simulink model "arithmetic"  (R2025a)
settings: Solver=FixedStepAuto  StartTime=0.0  StopTime=5  FixedStep=0.00001  MaxStep=0.001  RelTol=1e-3
values from neighbouring files (symbols this model uses):
  Fx = 600.0    [data.sldd]    (also in data2023.sldd)
  Fy = 800.0    [data.sldd]    (also in data2023.sldd)
  g = 10.0    [data.sldd]    (also in data2023.sldd)
  ma = 20.0    [data.sldd]    (also in data2023.sldd)
  mb = 50.0    [data.sldd]    (also in data2023.sldd)
  T0 = 500.0    [data.sldd]    (also in data2023.sldd = 20.0)
settings Model: DataDictionary=data.sldd  Creator=MangoJuice  LastModifiedBy=MangoJuice

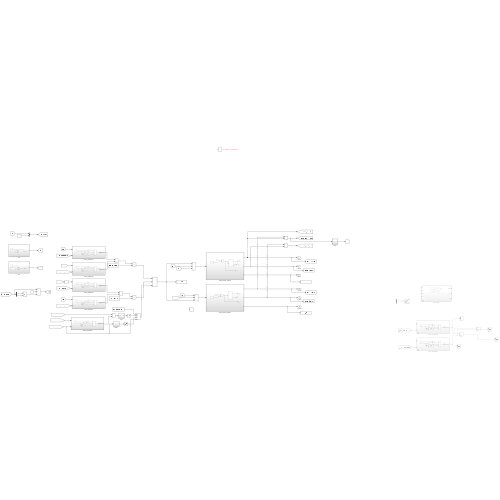
[thumbnail: Simulink's stored preview of the top-level diagram]
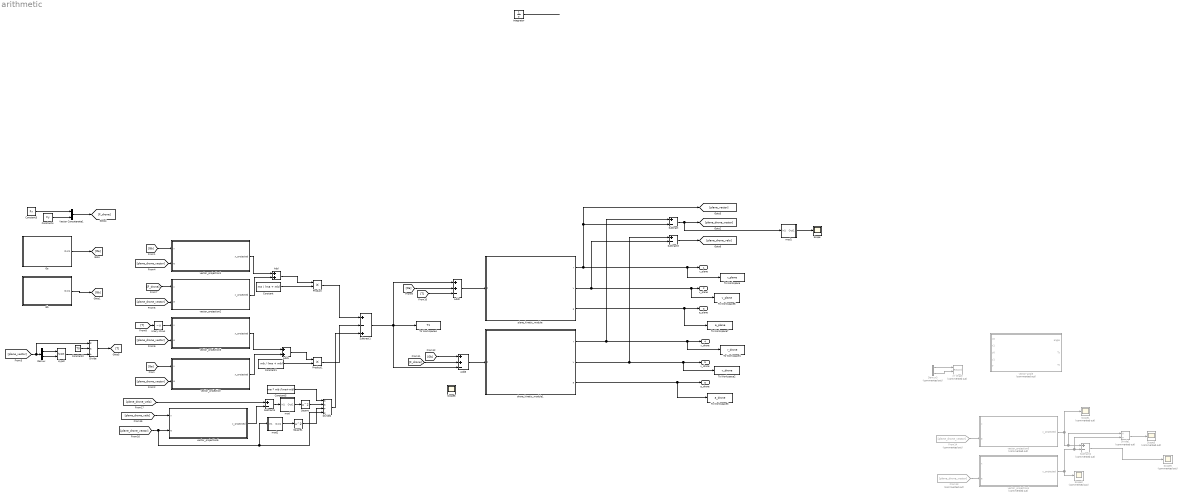
== system arithmetic ==
  Add : Sum
  Add1 : Sum
  Add2 : Sum  Inputs=++-
  Add3 : Sum  Inputs=++-
  Constant : Constant  Value=ma / (ma + mb)
  Constant1 : Constant  Value=mb / (ma + mb)
  Constant2 : Constant  Value=T0
  Constant3 : Constant  Value=Fx
  Constant4 : Constant  Value=Fy
  Constant5 : Constant  Value=ma * mb /(ma+mb)
  Demux : Demux  Outputs=2
  Demux3 : Demux  Commented=on  Outputs=2
  Divide : Product  Inputs=**/
  Divide1 : Product  Commented=on  Inputs=*/
  Divide2 : Product  Inputs=**/*
  From13 : From  Commented=on  GotoTag=plane_drone_vector
  From14 : From  Commented=on  GotoTag=plane_drone_vector
  Ga : Subsystem
  Gb : Subsystem
  Hypot : Math  Operator=hypot
  Integrator : Integrator
  Product : Product
  Product1 : Product
  Scope : Scope
      settings: ActiveDisplayYMinimum=49.999999999997144  ActiveDisplayYMaximum=50.0000000000041
  Scope{1..3,5} (4 alike) : Scope  Commented=on
      Scope1 settings: ActiveDisplayYMinimum=-1.094437041420969  ActiveDisplayYMaximum=6.4337390050976033
      Scope2 settings: ActiveDisplayYMinimum=-1  ActiveDisplayYMaximum=1  DataLoggingVariableName=ScopeData2
      Scope3 settings: ActiveDisplayYMinimum=-1.2740170172523153  ActiveDisplayYMaximum=0.9918630866201682  DataLoggingVariableName=ScopeData3
      Scope5 settings: ActiveDisplayYMinimum=-10.22400956516295  ActiveDisplayYMaximum=15.11556177661943  DataLoggingVariableName=ScopeData5
  Scope6 : Scope
      settings: ActiveDisplayYMinimum=99.999999999999943  ActiveDisplayYMaximum=100.00000000000006  DataLoggingVariableName=ScopeData6
  Square : Math  Operator=square
  Square1 : Math  Operator=square
  Subtract : Sum  Inputs=+-
  Subtract1 : Sum  Inputs=+-+
  Subtract2 : Sum  Commented=on  Inputs=+-
  Subtract3 : Sum  Inputs=+-
  Subtract4 : Sum  Inputs=+-
  To Workspace : ToWorkspace  VariableName=r_plane  SaveFormat=Timeseries  SampleTime=0.05
  To Workspace1 : ToWorkspace  VariableName=r_drone  SaveFormat=Timeseries  SampleTime=0.05
  To Workspace2 : ToWorkspace  VariableName=v_drone  SaveFormat=Timeseries  SampleTime=0.05
  To Workspace3 : ToWorkspace  VariableName=a_drone  SaveFormat=Timeseries  SampleTime=0.05
  To Workspace4 : ToWorkspace  VariableName=T1  SaveFormat=Timeseries  SampleTime=0.05
  To Workspace6 : ToWorkspace  VariableName=v_plane  SaveFormat=Timeseries  SampleTime=0.05
  To Workspace7 : ToWorkspace  VariableName=a_plane  SaveFormat=Timeseries  SampleTime=0.05
  Unary Minus : UnaryMinus
  Vector Concatenate1 : Concatenate
  XY Graph : Record  Commented=on  NumPorts=2.0  FileSettingsInternal="{\"entries\":[{\"content\":{\"excelSettings\":{\"content\":{},\"type\":\"Streamout.ExcelSettings\"},\"parquetSettings\":{\"content\":{},\"type\":\"Streamout.ParquetSettings\"}},\"type\":\"Streamout.FileSettingStorage\",\"uuid\":\"\"}],\"packageUris\":[\"http:\\/\\/schema.mathworks.com\\/mf0\\/streamout_blocks\\/R2020a\"],\"version\":\"1.0\"}"  FrameSettings=[0, 0]  Layout=[1 1]  SignalsInternal="{\"entries\":[{\"content\":{\"signals\":[{\"content\":{\"blockPath\":[],\"dimensions\":[1],\"domain\":\"\",\"lineColor\":\"#a2142f\",\"plots\":[ 1 ],\"port\":1,\"sid\":[\"\"],\"signalID\":1,\"signalName\":\"Demux3:1\"},\"type\":\"RecordBlkView.Signal\",\"uuid\":\"\"},{\"content\":{\"blockPath\":[],\"dimensions\":[1],\"domain\":\"\",\"lineColor\":\"#139fff\",\"plots\":[ 1 ],\"port\":2,\"sid\":[\"\"],\"signalID\":2,\"signalName\":\"Demux3:2\"},\"type\":\"RecordBlkView.Signal\",\"uuid\":\"\"}]},\"type\":\"RecordBlkView.InputSignals\",\"uuid\":\"\"}],\"packageUris\":[\"http:\\/\\/schema.mathworks.com\\/mf0\\/streamout_blocks\\/R2020a\"],\"version\":\"1.0\"}"  VisualizationBindings="{\"xyplotplugin\":{\"info\":[{\"series\":[{\"bindingParametersList\":[{\"parameter\":\"X-Axis\",\"signalID\":1,\"signalName\":\"Demux3:1\"},{\"parameter\":\"Y-Axis\",\"signalID\":2,\"signalName\":\"Demux3:2\"}],\"seriesID\":0}],\"subplotID\":1}]}}"  CompatibilityTag=XY
  drone_kinetic_module1 : Subsystem
  mod : Subsystem
  mod1 : Subsystem
  mod2 : Subsystem
  plane_kinetic_module : Subsystem
  vector-angle : Subsystem  Commented=on
  vector_projection : Subsystem
  vector_projection1 : Subsystem
  vector_projection2 : Subsystem
  vector_projection3 : Subsystem
  vector_projection4 : Subsystem  Commented=on
  vector_projection5 : Subsystem  Commented=on
  vector_projection6 : Subsystem
  r_plane : Outport
  v_plane : Outport  Port=2
  a_plane : Outport  Port=3
  r_drone : Outport  Port=4
  v_drone : Outport  Port=5
  a_drone : Outport  Port=6
  wires:
  Integrator/1 -> ?
  Ga/1(Out1) -> [Ga]
  Gb/1(Out1) -> [Gb]
  plane_kinetic_module/1(r) -> To Workspace/1, r_plane/1, [plane_vector], Subtract/2
  Subtract/1 -> mod1/1(In1), [plane_drone_vector]
  Hypot/1 -> Divide/3
  [plane_vector] -> Divide/1, Demux/1
  Demux/2 -> Hypot/2
  Demux/1 -> Hypot/1
  Constant2/1 -> Divide/2
  Vector Concatenate1/1 -> [F_drone]
  Constant3/1 -> Vector Concatenate1/1
  Constant4/1 -> Vector Concatenate1/2
  [Ga] -> vector_projection/1(x)
  [Gb] -> vector_projection1/1(x)
  [F_drone] -> vector_projection2/1(x)
  [plane_drone_vector] -> vector_projection/2(e)
  [plane_drone_vector] -> vector_projection1/2(e)
  [plane_drone_vector] -> vector_projection2/2(e)
  [plane_drone_vector] -> vector_projection3/2(e)
  vector_projection1/1(x_projected) -> Add/1
  vector_projection2/1(x_projected) -> Add/2
  Add/1 -> Product/1
  vector_projection3/1(x_projected) -> Add1/1
  vector_projection/1(x_projected) -> Add1/2
  Add1/1 -> Product1/1
  Product/1 -> Subtract1/1
  Product1/1 -> Subtract1/2
  Constant/1 -> Product/2
  Constant1/1 -> Product1/2
  Subtract1/1 -> To Workspace4/1, Add3/3, Add2/1
  Add2/1 -> plane_kinetic_module/1(F)
  [Ga] -> Add2/2
  [T] -> Add2/3
  Add3/1 -> drone_kinetic_module1/1(F)
  [F_drone] -> Add3/2
  [Gb] -> Add3/1
  vector_projection5/1(x_projected) -> Scope1/1, Divide1/1, Subtract2/1
  vector_projection4/1(x_projected) -> Scope2/1, Divide1/2, Subtract2/2
  From14/1 -> vector_projection5/2(e)
  From13/1 -> vector_projection4/2(e)
  Demux3/2 -> XY Graph/2
  Demux3/1 -> XY Graph/1
  Divide/1 -> [T]
  [T] -> Unary Minus/1
  Unary Minus/1 -> vector_projection3/1(x)
  Subtract2/1 -> Scope5/1
  Divide1/1 -> Scope3/1
  Subtract3/1 -> [plane_drone_velo]
  drone_kinetic_module1/2(v) -> To Workspace2/1, v_drone/1, Subtract3/1
  [plane_drone_velo] -> vector_projection6/1(x)
  vector_projection6/1(x_projected) -> Subtract4/2
  [plane_drone_velo] -> Subtract4/1
  Subtract4/1 -> mod/1(In1)
  mod/1(Out1) -> Square/1
  mod2/1(Out1) -> Square1/1
  [plane_drone_vector] -> Divide2/4, mod2/1(In1), vector_projection6/2(e)
  Square/1 -> Divide2/2
  Square1/1 -> Divide2/3
  Divide2/1 -> Subtract1/3
  Constant5/1 -> Divide2/1
  plane_kinetic_module/3(a) -> To Workspace7/1, a_plane/1
  drone_kinetic_module1/3(a) -> To Workspace3/1, a_drone/1
  plane_kinetic_module/2(v) -> To Workspace6/1, v_plane/1, Subtract3/2
  drone_kinetic_module1/1(r) -> To Workspace1/1, r_drone/1, Subtract/1
  mod1/1(Out1) -> Scope/1

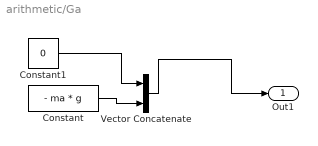
== system arithmetic/Ga ==
  Constant : Constant  Value=- ma * g  VectorParams1D=off
  Constant1 : Constant  Value=0
  Vector Concatenate : Concatenate
  Out1 : Outport
  wires:
  Constant1/1 -> Vector Concatenate/1
  Constant/1 -> Vector Concatenate/2
  Vector Concatenate/1 -> Out1/1

== system arithmetic/Gb ==
  Constant : Constant  Value=- mb * g  VectorParams1D=off
  Constant1 : Constant  Value=0
  Vector Concatenate : Concatenate
  Out1 : Outport
  wires:
  Vector Concatenate/1 -> Out1/1
  Constant/1 -> Vector Concatenate/2
  Constant1/1 -> Vector Concatenate/1

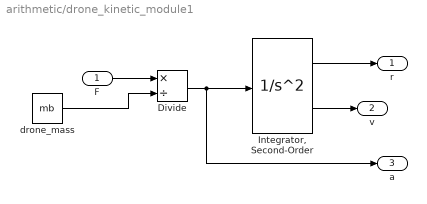
== system arithmetic/drone_kinetic_module1 ==
  F : Inport
  Divide : Product  Inputs=*/
  "Integrator, Second-Order" : SecondOrderIntegrator  ICX=drone_r0  ICDXDT=drone_v0
  drone_mass : Constant  Value=mb
  r : Outport
  v : Outport  Port=2
  a : Outport  Port=3
  wires:
  drone_mass/1 -> Divide/2
  "Integrator, Second-Order"/2 -> v/1
  "Integrator, Second-Order"/1 -> r/1
  Divide/1 -> a/1, "Integrator, Second-Order"/1
  F/1 -> Divide/1

== system arithmetic/mod ==
  In1 : Inport
  Demux4 : Demux  Outputs=2
  Hypot3 : Math  Operator=hypot
  Out1 : Outport
  wires:
  Demux4/1 -> Hypot3/1
  Demux4/2 -> Hypot3/2
  In1/1 -> Demux4/1
  Hypot3/1 -> Out1/1

== system arithmetic/mod1 ==
  In1 : Inport
  Demux4 : Demux  Outputs=2
  Hypot3 : Math  Operator=hypot
  Out1 : Outport
  wires:
  Demux4/1 -> Hypot3/1
  Demux4/2 -> Hypot3/2
  In1/1 -> Demux4/1
  Hypot3/1 -> Out1/1

== system arithmetic/mod2 ==
  In1 : Inport
  Demux4 : Demux  Outputs=2
  Hypot3 : Math  Operator=hypot
  Out1 : Outport
  wires:
  Hypot3/1 -> Out1/1
  In1/1 -> Demux4/1
  Demux4/2 -> Hypot3/2
  Demux4/1 -> Hypot3/1

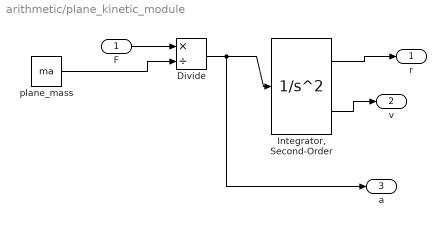
== system arithmetic/plane_kinetic_module ==
  F : Inport
  Divide : Product  Inputs=*/
  "Integrator, Second-Order" : SecondOrderIntegrator  ICX=plane_r0  ICDXDT=plane_v0
  plane_mass : Constant  Value=ma
  r : Outport
  v : Outport  Port=2
  a : Outport  Port=3
  wires:
  F/1 -> Divide/1
  Divide/1 -> a/1, "Integrator, Second-Order"/1
  "Integrator, Second-Order"/1 -> r/1
  "Integrator, Second-Order"/2 -> v/1
  plane_mass/1 -> Divide/2

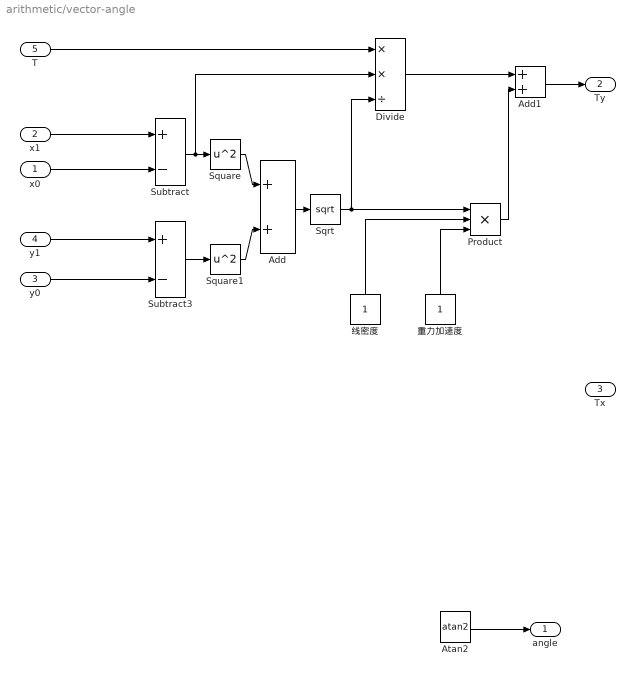
== system arithmetic/vector-angle ==
  x0 : Inport
  x1 : Inport  Port=2
  y0 : Inport  Port=3
  y1 : Inport  Port=4
  T : Inport  Port=5
  Add : Sum
  Add1 : Sum
  Atan2 : Trigonometry  Operator=atan2
  Divide : Product  Inputs=**/
  Product : Product  Inputs=3
  Sqrt : Sqrt
  Square : Math  Operator=square
  Square1 : Math  Operator=square
  Subtract : Sum  Inputs=+-
  Subtract3 : Sum  Inputs=+-
  线密度 : Constant
  重力加速度 : Constant
  angle : Outport
  Ty : Outport  Port=2
  Tx : Outport  Port=3
  wires:
  y0/1 -> Subtract3/2
  x1/1 -> Subtract/1
  Atan2/1 -> angle/1
  x0/1 -> Subtract/2
  y1/1 -> Subtract3/1
  Subtract/1 -> Divide/2, Square/1
  Subtract3/1 -> Square1/1
  Square/1 -> Add/1
  Square1/1 -> Add/2
  线密度/1 -> Product/2
  重力加速度/1 -> Product/3
  T/1 -> Divide/1
  Add/1 -> Sqrt/1
  Sqrt/1 -> Divide/3, Product/1
  Divide/1 -> Add1/1
  Product/1 -> Add1/2
  Add1/1 -> Ty/1

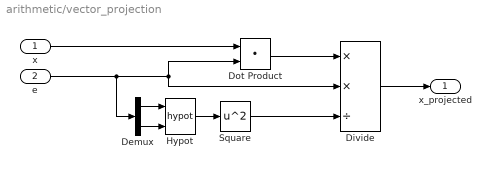
== system arithmetic/vector_projection ==
  x : Inport
  e : Inport  Port=2
  Demux : Demux  Outputs=2
  Divide : Product  Inputs=**/
  Dot Product : DotProduct  OutDataTypeStr=Inherit: Inherit via internal rule
  Hypot : Math  Operator=hypot
  Square : Math  Operator=square
  x_projected : Outport
  wires:
  x/1 -> Dot Product/1
  Divide/1 -> x_projected/1
  Hypot/1 -> Square/1
  e/1 -> Demux/1, Dot Product/2, Divide/2
  Demux/2 -> Hypot/2
  Demux/1 -> Hypot/1
  Square/1 -> Divide/3
  Dot Product/1 -> Divide/1

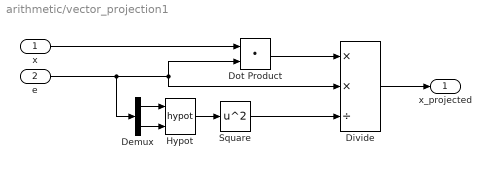
== system arithmetic/vector_projection1 ==
  x : Inport
  e : Inport  Port=2
  Demux : Demux  Outputs=2
  Divide : Product  Inputs=**/
  Dot Product : DotProduct  OutDataTypeStr=Inherit: Inherit via internal rule
  Hypot : Math  Operator=hypot
  Square : Math  Operator=square
  x_projected : Outport
  wires:
  Dot Product/1 -> Divide/1
  Square/1 -> Divide/3
  Demux/1 -> Hypot/1
  Demux/2 -> Hypot/2
  e/1 -> Divide/2, Dot Product/2, Demux/1
  Hypot/1 -> Square/1
  Divide/1 -> x_projected/1
  x/1 -> Dot Product/1

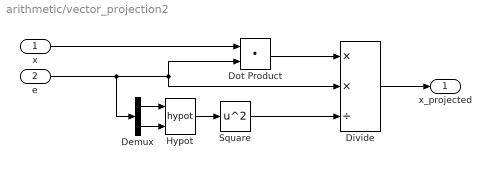
== system arithmetic/vector_projection2 ==
  x : Inport
  e : Inport  Port=2
  Demux : Demux  Outputs=2
  Divide : Product  Inputs=**/
  Dot Product : DotProduct  OutDataTypeStr=Inherit: Inherit via internal rule
  Hypot : Math  Operator=hypot
  Square : Math  Operator=square
  x_projected : Outport
  wires:
  x/1 -> Dot Product/1
  Divide/1 -> x_projected/1
  Hypot/1 -> Square/1
  e/1 -> Demux/1, Dot Product/2, Divide/2
  Demux/2 -> Hypot/2
  Demux/1 -> Hypot/1
  Square/1 -> Divide/3
  Dot Product/1 -> Divide/1

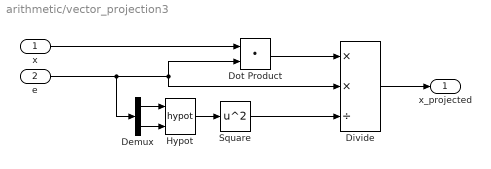
== system arithmetic/vector_projection3 ==
  x : Inport
  e : Inport  Port=2
  Demux : Demux  Outputs=2
  Divide : Product  Inputs=**/
  Dot Product : DotProduct  OutDataTypeStr=Inherit: Inherit via internal rule
  Hypot : Math  Operator=hypot
  Square : Math  Operator=square
  x_projected : Outport
  wires:
  Dot Product/1 -> Divide/1
  Square/1 -> Divide/3
  Demux/1 -> Hypot/1
  Demux/2 -> Hypot/2
  e/1 -> Divide/2, Dot Product/2, Demux/1
  Hypot/1 -> Square/1
  Divide/1 -> x_projected/1
  x/1 -> Dot Product/1

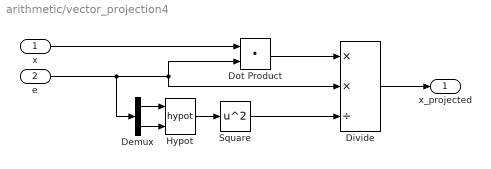
== system arithmetic/vector_projection4 ==
  x : Inport
  e : Inport  Port=2
  Demux : Demux  Outputs=2
  Divide : Product  Inputs=**/
  Dot Product : DotProduct  OutDataTypeStr=Inherit: Inherit via internal rule
  Hypot : Math  Operator=hypot
  Square : Math  Operator=square
  x_projected : Outport
  wires:
  Dot Product/1 -> Divide/1
  Square/1 -> Divide/3
  Demux/1 -> Hypot/1
  Demux/2 -> Hypot/2
  e/1 -> Divide/2, Dot Product/2, Demux/1
  Hypot/1 -> Square/1
  Divide/1 -> x_projected/1
  x/1 -> Dot Product/1

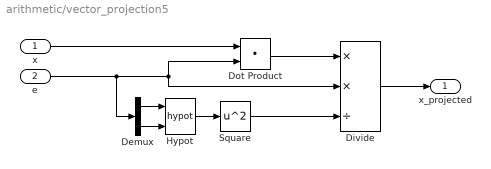
== system arithmetic/vector_projection5 ==
  x : Inport
  e : Inport  Port=2
  Demux : Demux  Outputs=2
  Divide : Product  Inputs=**/
  Dot Product : DotProduct  OutDataTypeStr=Inherit: Inherit via internal rule
  Hypot : Math  Operator=hypot
  Square : Math  Operator=square
  x_projected : Outport
  wires:
  x/1 -> Dot Product/1
  Divide/1 -> x_projected/1
  Hypot/1 -> Square/1
  e/1 -> Demux/1, Dot Product/2, Divide/2
  Demux/2 -> Hypot/2
  Demux/1 -> Hypot/1
  Square/1 -> Divide/3
  Dot Product/1 -> Divide/1

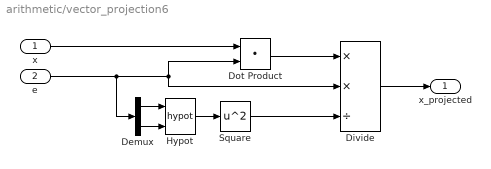
== system arithmetic/vector_projection6 ==
  x : Inport
  e : Inport  Port=2
  Demux : Demux  Outputs=2
  Divide : Product  Inputs=**/
  Dot Product : DotProduct  OutDataTypeStr=Inherit: Inherit via internal rule
  Hypot : Math  Operator=hypot
  Square : Math  Operator=square
  x_projected : Outport
  wires:
  Dot Product/1 -> Divide/1
  Square/1 -> Divide/3
  Demux/1 -> Hypot/1
  Demux/2 -> Hypot/2
  e/1 -> Divide/2, Dot Product/2, Demux/1
  Hypot/1 -> Square/1
  Divide/1 -> x_projected/1
  x/1 -> Dot Product/1
